simulink model "WindSpeedEstimator_sim"  (R2021b)
settings: Solver=FixedStepDiscrete  StartTime=0.0  StopTime=599.95  FixedStep=0.05  RelTol=1e-3
undefined symbols (not defined in the file or in its folder): dt, Parameter, v_0_est_0
libraries: simulink_need_slupdate x2, simulink x1
settings Model: Creator=david  LastModifiedBy=SchlipfSim

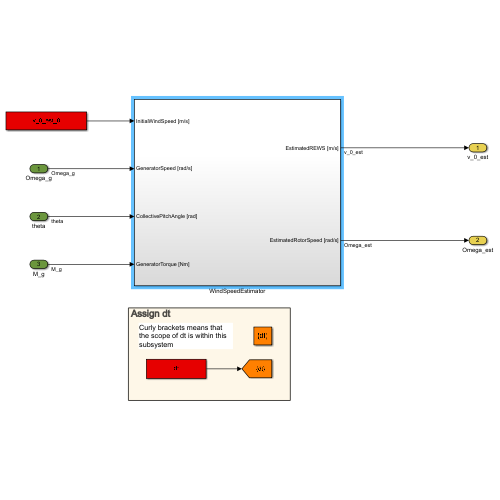
[thumbnail: Simulink's stored preview of the top-level diagram]
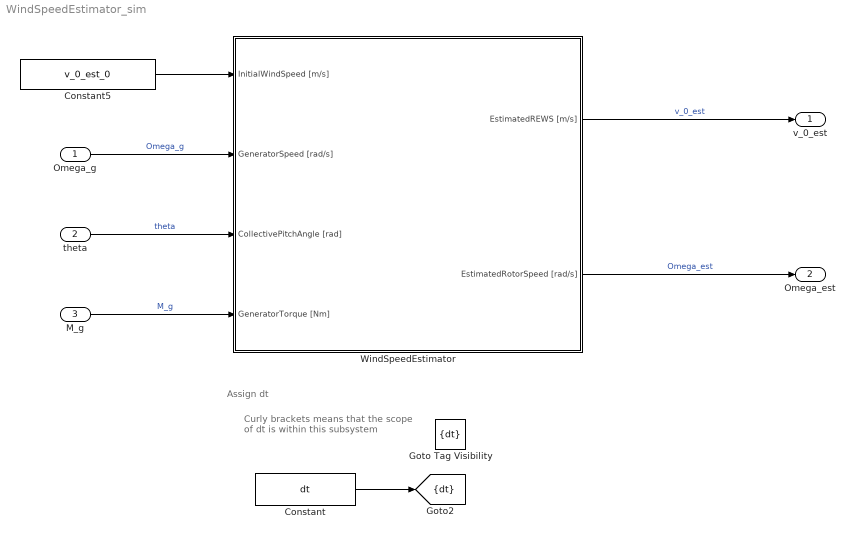
== system WindSpeedEstimator_sim ==
  note: Curly brackets means that the scope of dt is within this subsystem
  note: Assign dt
  Omega_g : Inport
  theta : Inport  Port=2
  M_g : Inport  Port=3
  Constant : Constant  Value=dt
  Constant5 : Constant  Value=v_0_est_0
  Goto Tag Visibility : GotoTagVisibility  GotoTag=dt
  WindSpeedEstimator : Subsystem
  v_0_est : Outport  VectorParamsAs1DForOutWhenUnconnected=off
  Omega_est : Outport  Port=2  VectorParamsAs1DForOutWhenUnconnected=off
  tag scope: dt=scoped
  wires:
  Constant5/1 -> WindSpeedEstimator/1(InitialWindSpeed [m/s])
  Constant/1 -> [dt]
  Omega_g/1 -> WindSpeedEstimator/2(GeneratorSpeed [rad/s])  "Omega_g"
  WindSpeedEstimator/1(EstimatedREWS [m/s]) -> v_0_est/1  "v_0_est"
  WindSpeedEstimator/2(EstimatedRotorSpeed [rad/s]) -> Omega_est/1  "Omega_est"
  theta/1 -> WindSpeedEstimator/3(CollectivePitchAngle [rad])  "theta"
  M_g/1 -> WindSpeedEstimator/4(GeneratorTorque [Nm])  "M_g"

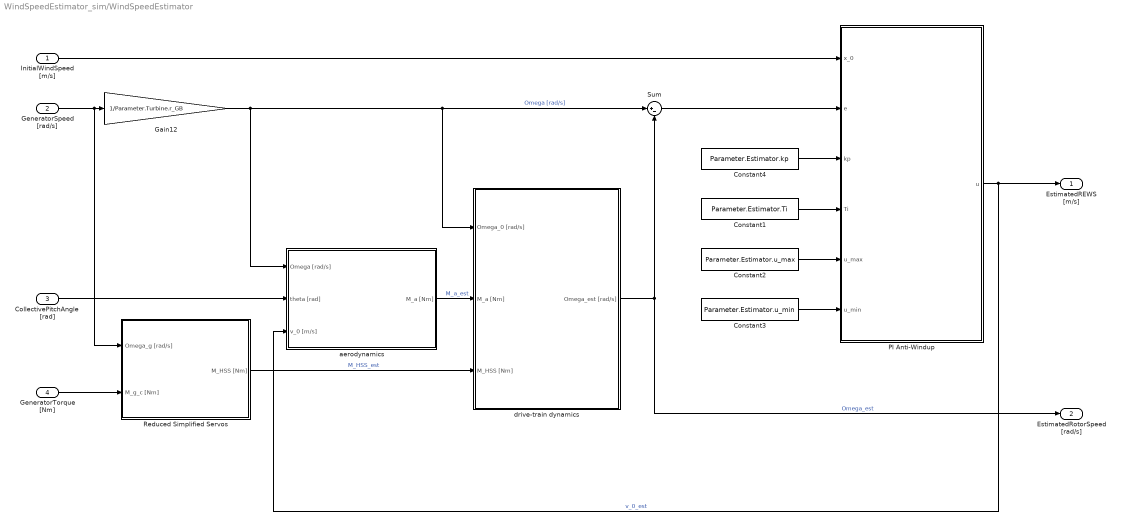
== system WindSpeedEstimator_sim/WindSpeedEstimator ==
  InitialWindSpeed [m/s] : Inport
  GeneratorSpeed [rad/s] : Inport  Port=2
  CollectivePitchAngle [rad] : Inport  Port=3
  GeneratorTorque [Nm] : Inport  Port=4
  Constant1 : Constant  Value=Parameter.Estimator.Ti
  Constant2 : Constant  Value=Parameter.Estimator.u_max
  Constant3 : Constant  Value=Parameter.Estimator.u_min
  Constant4 : Constant  Value=Parameter.Estimator.kp
  Gain12 : Gain  Gain=1/Parameter.Turbine.r_GB  SaturateOnIntegerOverflow=on  OutDataTypeStr=Inherit: Same as input  ParamDataTypeStr=Inherit: Same as input
  PI Anti-Windup : Subsystem
  Reduced Simplified Servos : Subsystem
  Sum : Sum  Inputs=|+-
  aerodynamics : Subsystem
  drive-train dynamics : Subsystem
  EstimatedREWS [m/s] : Outport
  EstimatedRotorSpeed [rad/s] : Outport  Port=2
  wires:
  Sum/1 -> PI Anti-Windup/2(e)
  Constant2/1 -> PI Anti-Windup/5(u_max)
  Gain12/1 -> aerodynamics/1(Omega [rad/s]), drive-train dynamics/1(Omega_0 [rad/s]), Sum/1  "Omega [rad/s]"
  Reduced Simplified Servos/1(M_HSS [Nm]) -> drive-train dynamics/3(M_HSS [Nm])  "M_HSS_est"
  drive-train dynamics/1(Omega_est [rad/s]) -> EstimatedRotorSpeed [rad/s]/1, Sum/2  "Omega_est"
  PI Anti-Windup/1(u) -> EstimatedREWS [m/s]/1, aerodynamics/3(v_0 [m/s])  "v_0_est"
  GeneratorSpeed [rad/s]/1 -> Reduced Simplified Servos/1(Omega_g [rad/s]), Gain12/1
  aerodynamics/1(M_a [Nm]) -> drive-train dynamics/2(M_a [Nm])  "M_a_est"
  Constant4/1 -> PI Anti-Windup/3(kp)
  Constant3/1 -> PI Anti-Windup/6(u_min)
  Constant1/1 -> PI Anti-Windup/4(Ti)
  InitialWindSpeed [m/s]/1 -> PI Anti-Windup/1(x_0)
  GeneratorTorque [Nm]/1 -> Reduced Simplified Servos/2(M_g_c [Nm])
  CollectivePitchAngle [rad]/1 -> aerodynamics/2(theta [rad])

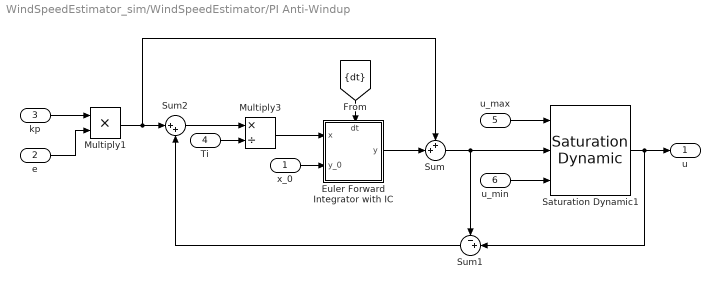
== system WindSpeedEstimator_sim/WindSpeedEstimator/PI Anti-Windup ==
  x_0 : Inport
  e : Inport  Port=2
  kp : Inport  Port=3
  Ti : Inport  Port=4
  u_max : Inport  Port=5
  u_min : Inport  Port=6
  Euler Forward Integrator with IC : Subsystem
      settings: PortSchema="{\"entries\":[{\"content\":{\"sides\":[{\"content\":{\"connectorIds\":[\"In1\",\"In2\"]},\"type\":\"ConnectorPlacement.EquallySpacedRectSide\",\"uuid\":\"2d8a7cce-2efd-4457-b68f-12cbbfaebd0c\"},{\"content\":{\"connectorIds\":[\"Out1\"],\"side\":\"RIGHT\"},\"type\":\"ConnectorPlacement.EquallySpacedRectSide\",\"uuid\":\"e0f9260e-921c-4bc7-b86b-28d84532dcd8\"},{\"content\":{\"connectorIds\":[\"In3\"],\"side\":\"TOP\"},\"type\":\"ConnectorPlacement.EquallySpacedRectSide\",\"uuid\":\"bc9e3329-6577-448f-99a1-0c4d852929dc\"}]},\"type\":\"ConnectorPlacement.EquallySpacedConnector\",\"uuid\":\"d9de99fe-6283-4a1f-aef3-e77ef8568bd4\"}],\"packageUris\":[\"http://schema.mathworks.com/mf0/Connector/R2020b\"],\"version\":\"1.0\"}"
      mask Display: disp("1\n-\ns")
  Multiply1 : Product  Inputs=**
  Multiply3 : Product  Inputs=*/
  Saturation Dynamic1 : simulink/Discontinuities/Saturation Dynamic  OutMin=[]  OutMax=[]  OutDataTypeStr=Inherit: Same as second input  OutDataType=fixdt(1, 16)  OutScaling=2^-10  DoSatur=off
  Sum : Sum  Inputs=++|
  Sum1 : Sum  Inputs=-+|
  Sum2 : Sum  Inputs=|++
  u : Outport  VectorParamsAs1DForOutWhenUnconnected=off
  wires:
  Saturation Dynamic1/1 -> u/1, Sum1/2
  kp/1 -> Multiply1/1
  e/1 -> Multiply1/2
  Ti/1 -> Multiply3/2
  Sum1/1 -> Sum2/2
  Multiply1/1 -> Sum/1, Sum2/1
  Sum2/1 -> Multiply3/1
  u_min/1 -> Saturation Dynamic1/3
  Sum/1 -> Saturation Dynamic1/2, Sum1/1
  u_max/1 -> Saturation Dynamic1/1
  [dt] -> Euler Forward Integrator with IC/3(dt)
  x_0/1 -> Euler Forward Integrator with IC/2(y_0)
  Euler Forward Integrator with IC/1(y) -> Sum/2
  Multiply3/1 -> Euler Forward Integrator with IC/1(x)

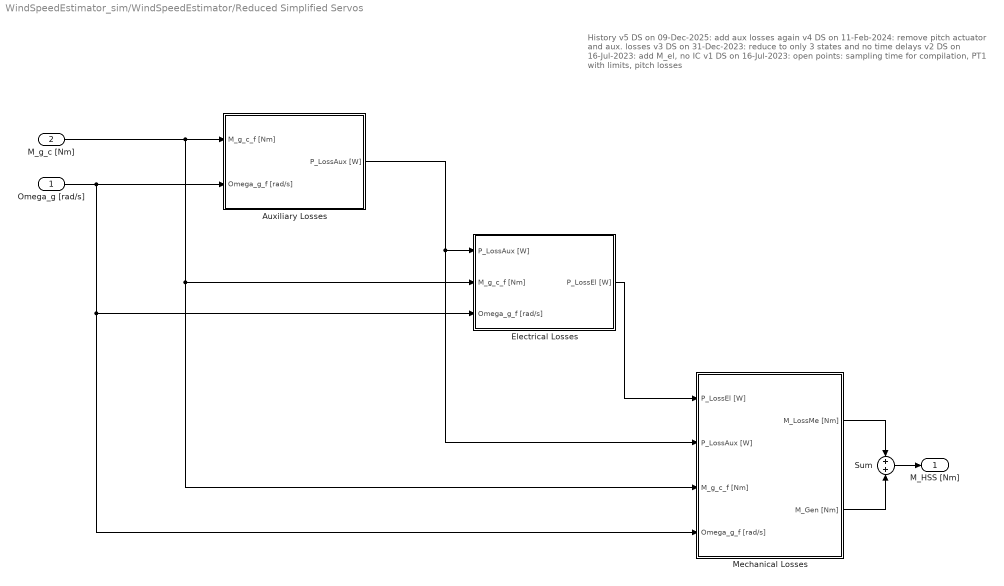
== system WindSpeedEstimator_sim/WindSpeedEstimator/Reduced Simplified Servos ==
  note: History
      | v5 DS on 09-Dec-2025: add aux losses again
      | v4 DS on 11-Feb-2024: remove pitch actuator and aux. losses
      | v3 DS on 31-Dec-2023: reduce to only 3 states and no time delays
      | v2 DS on 16-Jul-2023: add M_el, no IC
      | v1 DS on 16-Jul-2023: open points: sampling time for compilation, PT1 with limits, pitch losses
  Omega_g [rad/s] : Inport
  M_g_c [Nm] : Inport  Port=2
  Auxiliary Losses : Subsystem
  Electrical Losses : Subsystem
  Mechanical Losses : Subsystem
  Sum : Sum  Inputs=+|+
  M_HSS [Nm] : Outport
  wires:
  Auxiliary Losses/1(P_LossAux [W]) -> Electrical Losses/1(P_LossAux [W]), Mechanical Losses/2(P_LossAux [W])
  Mechanical Losses/2(M_Gen [Nm]) -> Sum/2
  Sum/1 -> M_HSS [Nm]/1
  Mechanical Losses/1(M_LossMe [Nm]) -> Sum/1
  Electrical Losses/1(P_LossEl [W]) -> Mechanical Losses/1(P_LossEl [W])
  Omega_g [rad/s]/1 -> Electrical Losses/3(Omega_g_f [rad/s]), Mechanical Losses/4(Omega_g_f [rad/s]), Auxiliary Losses/2(Omega_g_f [rad/s])
  M_g_c [Nm]/1 -> Electrical Losses/2(M_g_c_f [Nm]), Mechanical Losses/3(M_g_c_f [Nm]), Auxiliary Losses/1(M_g_c_f [Nm])

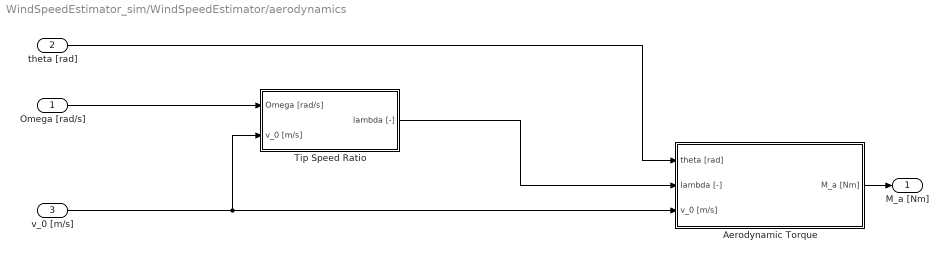
== system WindSpeedEstimator_sim/WindSpeedEstimator/aerodynamics ==
  Omega [rad/s] : Inport
  theta [rad] : Inport  Port=2
  v_0 [m/s] : Inport  Port=3
  Aerodynamic Torque : Subsystem
  Tip Speed Ratio : Subsystem
  M_a [Nm] : Outport  VectorParamsAs1DForOutWhenUnconnected=off
  wires:
  theta [rad]/1 -> Aerodynamic Torque/1(theta [rad])
  Aerodynamic Torque/1(M_a [Nm]) -> M_a [Nm]/1
  Omega [rad/s]/1 -> Tip Speed Ratio/1(Omega [rad/s])
  v_0 [m/s]/1 -> Aerodynamic Torque/3(v_0 [m/s]), Tip Speed Ratio/2(v_0 [m/s])
  Tip Speed Ratio/1(lambda [-]) -> Aerodynamic Torque/2(lambda [-])

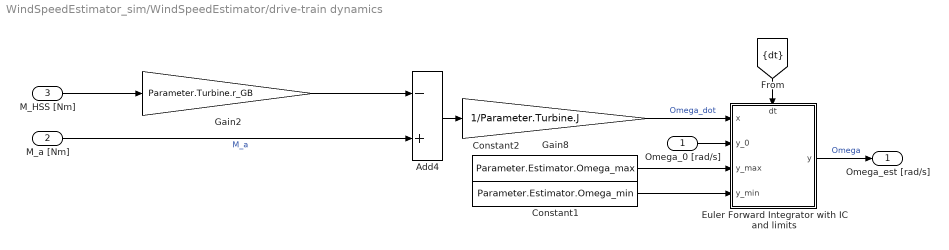
== system WindSpeedEstimator_sim/WindSpeedEstimator/drive-train dynamics ==
  Omega_0 [rad/s] : Inport
  M_a [Nm] : Inport  Port=2
  M_HSS [Nm] : Inport  Port=3
  Add4 : Sum  Inputs=-+
  Constant1 : Constant  Value=Parameter.Estimator.Omega_min
  Constant2 : Constant  Value=Parameter.Estimator.Omega_max
  Euler Forward Integrator with IC and limits : Subsystem
      settings: PortSchema="{\"entries\":[{\"content\":{\"sides\":[{\"content\":{\"connectorIds\":[\"In1\",\"In2\",\"In3\",\"In4\"]},\"type\":\"ConnectorPlacement.EquallySpacedRectSide\",\"uuid\":\"2d8a7cce-2efd-4457-b68f-12cbbfaebd0c\"},{\"content\":{\"connectorIds\":[\"Out1\"],\"side\":\"RIGHT\"},\"type\":\"ConnectorPlacement.EquallySpacedRectSide\",\"uuid\":\"e0f9260e-921c-4bc7-b86b-28d84532dcd8\"},{\"content\":{\"connectorIds\":[\"In5\"],\"side\":\"TOP\"},\"type\":\"ConnectorPlacement.EquallySpacedRectSide\",\"uuid\":\"bc9e3329-6577-448f-99a1-0c4d852929dc\"}]},\"type\":\"ConnectorPlacement.EquallySpacedConnector\",\"uuid\":\"d9de99fe-6283-4a1f-aef3-e77ef8568bd4\"}],\"packageUris\":[\"http://schema.mathworks.com/mf0/Connector/R2020b\"],\"version\":\"1.0\"}"
      mask Display: disp("1\n-\ns")
  Gain2 : Gain  Gain=Parameter.Turbine.r_GB  SaturateOnIntegerOverflow=on  OutDataTypeStr=Inherit: Same as input  ParamDataTypeStr=Inherit: Same as input
  Gain8 : Gain  Gain=1/Parameter.Turbine.J  SaturateOnIntegerOverflow=on  OutDataTypeStr=Inherit: Same as input  ParamDataTypeStr=Inherit: Same as input
  Omega_est [rad/s] : Outport  VectorParamsAs1DForOutWhenUnconnected=off
  wires:
  M_a [Nm]/1 -> Add4/2  "M_a"
  Add4/1 -> Gain8/1
  Gain8/1 -> Euler Forward Integrator with IC and limits/1(x)  "Omega_dot"
  Gain2/1 -> Add4/1
  Euler Forward Integrator with IC and limits/1(y) -> Omega_est [rad/s]/1  "Omega"
  M_HSS [Nm]/1 -> Gain2/1
  Omega_0 [rad/s]/1 -> Euler Forward Integrator with IC and limits/2(y_0)
  [dt] -> Euler Forward Integrator with IC and limits/5(dt)
  Constant2/1 -> Euler Forward Integrator with IC and limits/3(y_max)
  Constant1/1 -> Euler Forward Integrator with IC and limits/4(y_min)

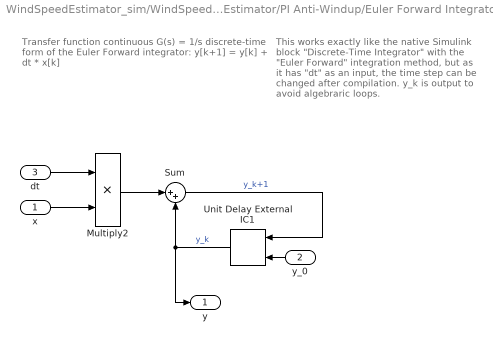
== system WindSpeedEstimator_sim/WindSpeedEstimator/PI Anti-Windup/Euler Forward Integrator with IC ==
  note: This works exactly like the native Simulink block "Discrete-Time Integrator" with the "Euler Forward" integration method, but as it has "dt" as an input, the time step can be changed after compilation.
      | y_k is output to avoid algebraric loops.
  note: Transfer function continuous
      |
      | G(s) = 1/s
      |
      | discrete-time form of the Euler Forward integrator:
      |
      | y[k+1] = y[k] + dt * x[k]
  x : Inport
  y_0 : Inport  Port=2
  dt : Inport  Port=3
  Multiply2 : Product  Inputs=**
  Sum : Sum  Inputs=|++
  Unit Delay External IC1 : simulink_need_slupdate/Unit Delay External IC  tsamp=-1
      settings: SourceProductBaseCode=SL
  y : Outport  VectorParamsAs1DForOutWhenUnconnected=off
  wires:
  dt/1 -> Multiply2/1
  Sum/1 -> Unit Delay External IC1/1  "y_k+1"
  Multiply2/1 -> Sum/1
  Unit Delay External IC1/1 -> Sum/2, y/1  "y_k"
  y_0/1 -> Unit Delay External IC1/2
  x/1 -> Multiply2/2

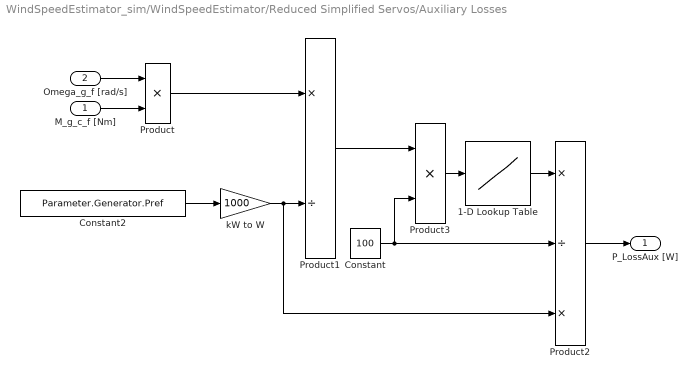
== system WindSpeedEstimator_sim/WindSpeedEstimator/Reduced Simplified Servos/Auxiliary Losses ==
  M_g_c_f [Nm] : Inport
  Omega_g_f [rad/s] : Inport  Port=2
  1-D Lookup Table : Lookup_n-D  NumberOfTableDimensions=1  BreakpointsForDimension1=Parameter.Generator.AuxLossTable.x  Table=Parameter.Generator.AuxLossTable.y  ExtrapMethod=Clip  UseLastTableValue=on  InternalRulePriority=Speed  RndMeth=Simplest  InputSameDT=on
  Constant : Constant  Value=100
  Constant2 : Constant  Value=Parameter.Generator.Pref
  Product : Product
  Product1 : Product  Inputs=*/
  Product2 : Product  Inputs=*/*
  Product3 : Product
  kW to W : Gain  Gain=1000
  P_LossAux [W] : Outport  VectorParamsAs1DForOutWhenUnconnected=off
  wires:
  M_g_c_f [Nm]/1 -> Product/2
  Omega_g_f [rad/s]/1 -> Product/1
  Product/1 -> Product1/1
  1-D Lookup Table/1 -> Product2/1
  Constant/1 -> Product3/2, Product2/2
  Product2/1 -> P_LossAux [W]/1
  Product3/1 -> 1-D Lookup Table/1
  Product1/1 -> Product3/1
  Constant2/1 -> kW to W/1
  kW to W/1 -> Product2/3, Product1/2

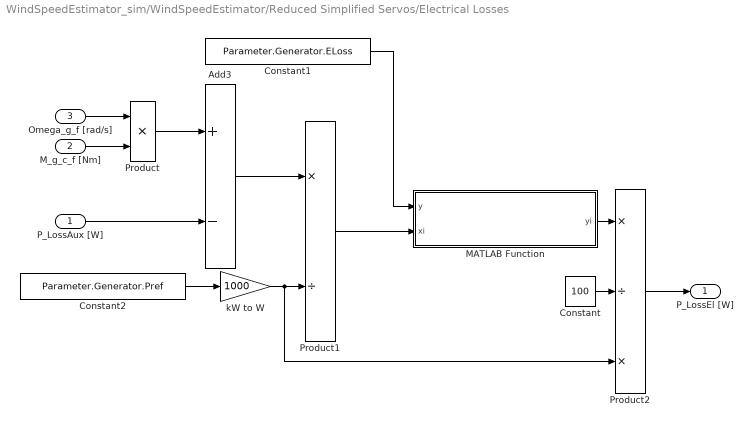
== system WindSpeedEstimator_sim/WindSpeedEstimator/Reduced Simplified Servos/Electrical Losses ==
  P_LossAux [W] : Inport
  M_g_c_f [Nm] : Inport  Port=2
  Omega_g_f [rad/s] : Inport  Port=3
  Add3 : Sum  Inputs=+-
  Constant : Constant  Value=100
  Constant1 : Constant  Value=Parameter.Generator.ELoss
  Constant2 : Constant  Value=Parameter.Generator.Pref
  MATLAB Function : MATLAB Function  TreatAsAtomicUnit=on
  Product : Product
  Product1 : Product  Inputs=*/
  Product2 : Product  Inputs=*/*
  kW to W : Gain  Gain=1000
  P_LossEl [W] : Outport  VectorParamsAs1DForOutWhenUnconnected=off
  wires:
  Product/1 -> Add3/1
  Omega_g_f [rad/s]/1 -> Product/1
  M_g_c_f [Nm]/1 -> Product/2
  P_LossAux [W]/1 -> Add3/2
  Add3/1 -> Product1/1
  Constant/1 -> Product2/2
  Product2/1 -> P_LossEl [W]/1
  MATLAB Function/1(yi) -> Product2/1
  Product1/1 -> MATLAB Function/2(xi)
  Constant1/1 -> MATLAB Function/1(y)
  Constant2/1 -> kW to W/1
  kW to W/1 -> Product2/3, Product1/2

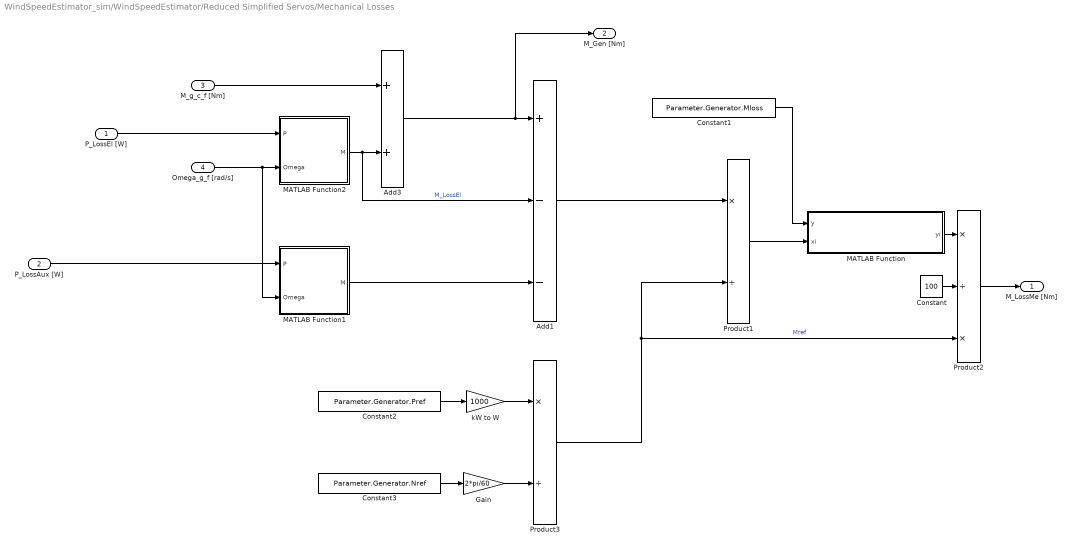
== system WindSpeedEstimator_sim/WindSpeedEstimator/Reduced Simplified Servos/Mechanical Losses ==
  P_LossEl [W] : Inport
  P_LossAux [W] : Inport  Port=2
  M_g_c_f [Nm] : Inport  Port=3
  Omega_g_f [rad/s] : Inport  Port=4
  Add1 : Sum  Inputs=+--
  Add3 : Sum
  Constant : Constant  Value=100
  Constant1 : Constant  Value=Parameter.Generator.Mloss
  Constant2 : Constant  Value=Parameter.Generator.Pref
  Constant3 : Constant  Value=Parameter.Generator.Nref
  Gain : Gain  Gain=2*pi/60
  MATLAB Function : MATLAB Function  TreatAsAtomicUnit=on
  MATLAB Function1 : MATLAB Function  TreatAsAtomicUnit=on
  MATLAB Function2 : MATLAB Function  TreatAsAtomicUnit=on
  Product1 : Product  Inputs=*/
  Product2 : Product  Inputs=*/*
  Product3 : Product  Inputs=*/
  kW to W : Gain  Gain=1000
  M_LossMe [Nm] : Outport  VectorParamsAs1DForOutWhenUnconnected=off
  M_Gen [Nm] : Outport  Port=2  VectorParamsAs1DForOutWhenUnconnected=off
  wires:
  Constant1/1 -> MATLAB Function/1(y)
  Product1/1 -> MATLAB Function/2(xi)
  MATLAB Function/1(yi) -> Product2/1
  Product2/1 -> M_LossMe [Nm]/1
  Constant/1 -> Product2/2
  M_g_c_f [Nm]/1 -> Add3/1
  Constant2/1 -> kW to W/1
  Constant3/1 -> Gain/1
  Gain/1 -> Product3/2
  Product3/1 -> Product2/3, Product1/2  "Mref"
  MATLAB Function2/1(M) -> Add1/2, Add3/2  "M_LossEl"
  Add3/1 -> M_Gen [Nm]/1, Add1/1
  Add1/1 -> Product1/1
  P_LossAux [W]/1 -> MATLAB Function1/1(P)
  MATLAB Function1/1(M) -> Add1/3
  P_LossEl [W]/1 -> MATLAB Function2/1(P)
  Omega_g_f [rad/s]/1 -> MATLAB Function1/2(Omega), MATLAB Function2/2(Omega)
  kW to W/1 -> Product3/1

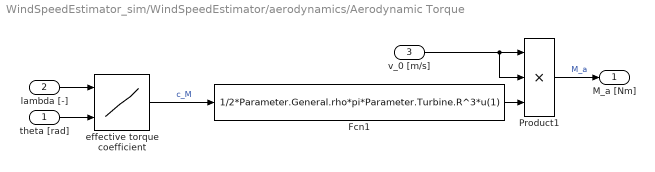
== system WindSpeedEstimator_sim/WindSpeedEstimator/aerodynamics/Aerodynamic Torque ==
  theta [rad] : Inport
  lambda [-] : Inport  Port=2
  v_0 [m/s] : Inport  Port=3
  Fcn1 : Fcn  Expr=1/2*Parameter.General.rho*pi*Parameter.Turbine.R^3*u(1)
  Product1 : Product  Inputs=3  RndMeth=Zero
  effective torque coefficient : Lookup2D  RowIndex=Parameter.Turbine.SS.lambda  ColumnIndex=Parameter.Turbine.SS.theta  Table=Parameter.Turbine.SS.c_M  LookUpMeth=Interpolation-Use End Values
  M_a [Nm] : Outport  VectorParamsAs1DForOutWhenUnconnected=off
  wires:
  Product1/1 -> M_a [Nm]/1  "M_a"
  Fcn1/1 -> Product1/3
  lambda [-]/1 -> effective torque coefficient/1
  theta [rad]/1 -> effective torque coefficient/2
  v_0 [m/s]/1 -> Product1/1, Product1/2
  effective torque coefficient/1 -> Fcn1/1  "c_M"

== system WindSpeedEstimator_sim/WindSpeedEstimator/aerodynamics/Tip Speed Ratio ==
  Omega [rad/s] : Inport
  v_0 [m/s] : Inport  Port=2
  Gain6 : Gain  Gain=Parameter.Turbine.R  SaturateOnIntegerOverflow=on  OutDataTypeStr=Inherit: Same as input  ParamDataTypeStr=Inherit: Same as input
  Product3 : Product  Inputs=*/  RndMeth=Zero
  lambda [-] : Outport  VectorParamsAs1DForOutWhenUnconnected=off
  wires:
  Product3/1 -> Gain6/1
  Omega [rad/s]/1 -> Product3/1
  v_0 [m/s]/1 -> Product3/2
  Gain6/1 -> lambda [-]/1  "lambda"

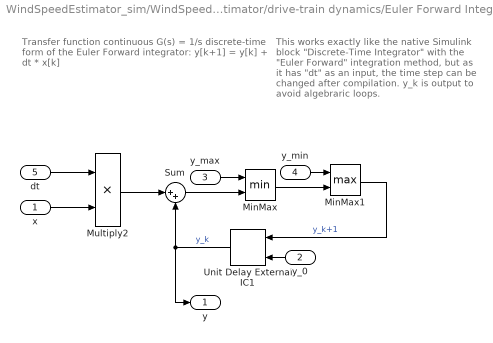
== system WindSpeedEstimator_sim/WindSpeedEstimator/drive-train dynamics/Euler Forward Integrator with IC and limits ==
  note: This works exactly like the native Simulink block "Discrete-Time Integrator" with the "Euler Forward" integration method, but as it has "dt" as an input, the time step can be changed after compilation.
      | y_k is output to avoid algebraric loops.
  note: Transfer function continuous
      |
      | G(s) = 1/s
      |
      | discrete-time form of the Euler Forward integrator:
      |
      | y[k+1] = y[k] + dt * x[k]
  x : Inport
  y_0 : Inport  Port=2
  y_max : Inport  Port=3
  y_min : Inport  Port=4
  dt : Inport  Port=5
  MinMax : MinMax  Inputs=2
  MinMax1 : MinMax  Function=max  Inputs=2
  Multiply2 : Product  Inputs=**
  Sum : Sum  Inputs=|++
  Unit Delay External IC1 : simulink_need_slupdate/Unit Delay External IC  tsamp=-1
      settings: SourceProductBaseCode=SL
  y : Outport  VectorParamsAs1DForOutWhenUnconnected=off
  wires:
  dt/1 -> Multiply2/1
  Multiply2/1 -> Sum/1
  Unit Delay External IC1/1 -> Sum/2, y/1  "y_k"
  y_0/1 -> Unit Delay External IC1/2
  x/1 -> Multiply2/2
  Sum/1 -> MinMax/2
  MinMax/1 -> MinMax1/2
  MinMax1/1 -> Unit Delay External IC1/1  "y_k+1"
  y_min/1 -> MinMax1/1
  y_max/1 -> MinMax/1

== matlab function WindSpeedEstimator_sim/WindSpeedEstimator/Reduced Simplified Servos/Mechanical Losses/MATLAB Function ==
  data: y input; yi output; xi input
function yi = NewtonQuadraticInterpolation(y,xi)
% https://pythonnumericalmethods.berkeley.edu/notebooks/chapter17.05-Newtons-Polynomial-Interpolation.html
% https://www.lernhelfer.de/schuelerlexikon/mathematik-abitur/artikel/newtonsches-und-lagrangesches-interpolationsverfahren#
% with x0=0; x1=1/2; x2=1;

% coefficients
y0 = y(1);
y1 = y(2);
y2 = y(3);
a0 =                 y0;    % y0 = a0
a1 =        2*y1 - 2*y0;    % y1 = a0 + a1*(x1-x0)                      = a0 + a1*1/2
a2 = 2*y2 - 4*y1 + 2*y0;    % y2 = a0 + a1*(x2-x0) + a2*(x2-x0)*(x2-x1) = a0 + a1     + a2*1/2

% polynomial
% p(x) = a0 + a1*(x-x0) + a2*(x-x0)*(x-x1)
% p(x) = a0 + (a1-1/2*a2)*x + a2*x^2
p0 = a0;                    
p1 = a1-1/2*a2;
p2 = a2;

% interpolation
yi = p0 + p1 * xi + p2 * xi.^2;

end

== matlab function WindSpeedEstimator_sim/WindSpeedEstimator/Reduced Simplified Servos/Mechanical Losses/MATLAB Function1 ==
  data: P input; M output; Omega input
function M = RobustTorque(P,Omega)

epsilon = 1e-10;

if abs(Omega)>epsilon
    M = P/Omega;
else
    M = 0;
end

end

== matlab function WindSpeedEstimator_sim/WindSpeedEstimator/Reduced Simplified Servos/Mechanical Losses/MATLAB Function2 ==
  data: P input; M output; Omega input
function M = RobustTorque(P,Omega)

epsilon = 1e-10;

if abs(Omega)>epsilon
    M = P/Omega;
else
    M = 0;
end

end

== matlab function WindSpeedEstimator_sim/WindSpeedEstimator/Reduced Simplified Servos/Electrical Losses/MATLAB Function ==
  data: y input; yi output; xi input
function yi = NewtonQuadraticInterpolation(y,xi)
% https://pythonnumericalmethods.berkeley.edu/notebooks/chapter17.05-Newtons-Polynomial-Interpolation.html
% https://www.lernhelfer.de/schuelerlexikon/mathematik-abitur/artikel/newtonsches-und-lagrangesches-interpolationsverfahren#
% with x0=0; x1=1/2; x2=1;

% coefficients
y0 = y(1);
y1 = y(2);
y2 = y(3);
a0 =                 y0;    % y0 = a0
a1 =        2*y1 - 2*y0;    % y1 = a0 + a1*(x1-x0)                      = a0 + a1*1/2
a2 = 2*y2 - 4*y1 + 2*y0;    % y2 = a0 + a1*(x2-x0) + a2*(x2-x0)*(x2-x1) = a0 + a1     + a2*1/2

% polynomial
% p(x) = a0 + a1*(x-x0) + a2*(x-x0)*(x-x1)
% p(x) = a0 + (a1-1/2*a2)*x + a2*x^2
p0 = a0;                    
p1 = a1-1/2*a2;
p2 = a2;

% interpolation
yi = p0 + p1 * xi + p2 * xi.^2;

end
